simulink model "AnalysisSimAP"  (R2016a)
settings: Solver=VariableStepAuto  StartTime=0.0  StopTime=5  RelTol=1e-3
values from neighbouring files (symbols this model uses):
  C = -C*[1, -1]    [RobustnessAnalysisAP.m]    (also in RobustnessAnalysis_MIL9490.m = -[1; 1]*C*[1, -1])
  GeriFDsysPID2_IO = NdofwActSens(okeep,ikeep,AEC6,ModeShape,FEM,Vmps,aeroProp,massProp,     coeffdataPIDfull,actdata,sensdata)    [GenerateGeriModelAP.m]    (also in RobustnessAnalysisAP.m = P; RobustnessAnalysis_MIL9490.m = P)
  Vinf = Vinfs    [RobustnessAnalysisAP.m]    (also in RobustnessAnalysis_MIL9490.m; example_geri.mat = [25 26 27 28 29 30 31 32 33 34 35 36 ... (21 elements, 1x21))
undefined symbols (not defined in the file or in its folder): K
libraries: simulink_extras x7, cstblocks x5, dspsigattribs x4
settings Model: Creator=Julian  LastModifiedBy=juliant
settings GRTTargetCC: GeneratePreprocessorConditionals=Use local settings

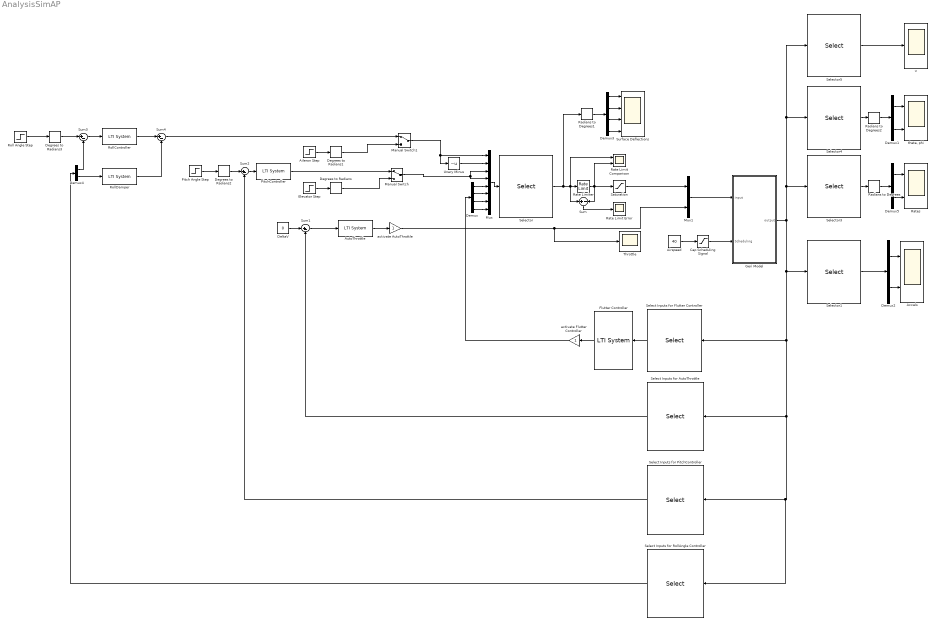
== system AnalysisSimAP ==
  Accels : Scope  NumInputPorts=2
  Aileron Step : Step  Time=3  After=0  SampleTime=0
  Airspeed : Constant  Value=40
  AutoThrottle : cstblocks/LTI System  sys=AutoThrottle  IC=[]
  Cap Scheduling Signal : Saturate  UpperLimit=45  LowerLimit=25
  Degrees to Radians{,1..3} (4 alike) : simulink_extras/Transformations/Degrees to Radians
  DeltaV : Constant  Value=0
  Demux : Demux  Outputs=[1 1 1 1]
  Demux1 : Demux  Outputs=2
  Demux2 : Demux  Outputs=[3 3]
  Demux3 : Demux  Outputs=[2 2 2 2]
  Demux4 : Demux  Outputs=2
  Demux5 : Demux  Outputs=2
  Elevator Step : Step  SampleTime=0
  Flutter Controller : cstblocks/LTI System  sys=-C  IC=[]
  Geri Model : Subsystem
  Manual Switch : ManualSwitch
  Manual Switch1 : ManualSwitch
  Mux : Mux  Inputs=8
  Mux1 : Mux  Inputs=[8 1]
  Pitch Angle Step : Step  Time=0.5  After=10  SampleTime=0
  PitchController : cstblocks/LTI System  sys=PitchController  IC=[]
  Radians to Degrees : simulink_extras/Transformations/Radians to Degrees
  Radians to Degrees1 : simulink_extras/Transformations/Radians to Degrees
  Radians to Degrees2 : simulink_extras/Transformations/Radians to Degrees
  Rate Limit Comparison : Scope  NumInputPorts=2
  Rate Limit Error : Scope
  Rate Limiter : RateLimiter  RisingSlewLimit=30/180*pi  FallingSlewLimit=-30/180*pi  SampleTimeMode=inherited
  Rates : Scope  NumInputPorts=2
  Roll Angle Step : Step  Time=2  After=20  SampleTime=0
  RollController : cstblocks/LTI System  sys=RollController  IC=[]
  RollDamper : cstblocks/LTI System  sys=RollDamper  IC=[]
  Saturation : Saturate  UpperLimit=30/180*pi  LowerLimit=-30/180*pi
  Select Inputs for AutoThrottle : Selector  InputPortWidth=11  IndexOptions=Index vector (dialog)  Indices=1  OutputSizes=1
  Select Inputs for Flutter Controller : Selector  InputPortWidth=11  IndexOptions=Index vector (dialog)  Indices=4:11  OutputSizes=1
  Select Inputs for PitchController : Selector  InputPortWidth=11  IndexOptions=Index vector (dialog)  Indices=2  OutputSizes=1
  Select Inputs for RollAngle Controller : Selector  InputPortWidth=11  IndexOptions=Index vector (dialog)  Indices=[3 5]  OutputSizes=1
  Selector : Selector  InputPortWidth=8  IndexOptions=Index vector (dialog)  Indices=[5 6 1 2 3 4 7 8]  OutputSizes=1
  Selector1 : Selector  InputPortWidth=11  IndexOptions=Index vector (dialog)  Indices=[11 7 10 9 6 8]  OutputSizes=1
  Selector3 : Selector  InputPortWidth=11  IndexOptions=Index vector (dialog)  Indices=[4 5]  OutputSizes=1
  Selector4 : Selector  InputPortWidth=11  IndexOptions=Index vector (dialog)  Indices=[2 3]  OutputSizes=1
  Selector5 : Selector  InputPortWidth=11  IndexOptions=Index vector (dialog)  Indices=[1]  OutputSizes=1
  Sum : Sum  Inputs=+-
  Sum{1..4} (4 alike) : Sum  Inputs=|+-
  Surface Deflections : Scope  NumInputPorts=4
  Throttle : Scope
  Unary Minus : UnaryMinus
  activate AutoThrottle : Gain
  activate Flutter Controller : Gain
  "theta, phi" : Scope  NumInputPorts=2
  u : Scope
  wires:
  Cap Scheduling Signal/1 -> Geri Model/2(Scheduling)
  Airspeed/1 -> Cap Scheduling Signal/1
  Mux/1 -> Selector/1
  Flutter Controller/1 -> activate Flutter Controller/1
  Demux/4 -> Mux/8
  Demux/3 -> Mux/7
  Demux/2 -> Mux/6
  Demux/1 -> Mux/5
  Manual Switch/1 -> Mux/3, Mux/4
  Aileron Step/1 -> Degrees to Radians1/1
  Manual Switch1/1 -> Mux/1, Unary Minus/1
  Selector3/1 -> Radians to Degrees/1
  Geri Model/1(output) -> Selector5/1, Selector4/1, Selector3/1, Selector1/1, Select Inputs for RollAngle Controller/1, Select Inputs for PitchController/1, Select Inputs for AutoThrottle/1, Select Inputs for Flutter Controller/1
  Selector1/1 -> Demux2/1
  Demux2/1 -> Accels/1
  Demux2/2 -> Accels/2
  activate Flutter Controller/1 -> Demux/1
  Radians to Degrees/1 -> Demux5/1
  Radians to Degrees1/1 -> Demux3/1
  Demux3/1 -> Surface Deflections/1
  Demux3/3 -> Surface Deflections/3
  Demux3/2 -> Surface Deflections/2
  Demux3/4 -> Surface Deflections/4
  Saturation/1 -> Mux1/1
  Rate Limiter/1 -> Saturation/1, Sum/2, Rate Limit Comparison/2
  Sum/1 -> Rate Limit Error/1
  Select Inputs for Flutter Controller/1 -> Flutter Controller/1
  AutoThrottle/1 -> activate AutoThrottle/1
  Select Inputs for AutoThrottle/1 -> Sum1/2
  Sum1/1 -> AutoThrottle/1
  DeltaV/1 -> Sum1/1
  Elevator Step/1 -> Degrees to Radians/1
  Pitch Angle Step/1 -> Degrees to Radians2/1
  Sum2/1 -> PitchController/1
  Select Inputs for PitchController/1 -> Sum2/2
  PitchController/1 -> Manual Switch/1
  Sum4/1 -> Manual Switch1/1
  Sum3/1 -> RollController/1
  Roll Angle Step/1 -> Degrees to Radians3/1
  Select Inputs for RollAngle Controller/1 -> Demux4/1
  Degrees to Radians1/1 -> Manual Switch1/2
  Degrees to Radians/1 -> Manual Switch/2
  Degrees to Radians2/1 -> Sum2/1
  Degrees to Radians3/1 -> Sum3/1
  RollController/1 -> Sum4/1
  RollDamper/1 -> Sum4/2
  Demux4/2 -> RollDamper/1
  Demux4/1 -> Sum3/2
  Selector/1 -> Radians to Degrees1/1, Sum/1, Rate Limit Comparison/1, Rate Limiter/1
  Radians to Degrees2/1 -> Demux1/1
  Selector4/1 -> Radians to Degrees2/1
  Selector5/1 -> u/1
  Demux1/1 -> "theta, phi"/1
  Demux1/2 -> "theta, phi"/2
  Demux5/1 -> Rates/1
  Demux5/2 -> Rates/2
  Unary Minus/1 -> Mux/2
  activate AutoThrottle/1 -> Throttle/1, Mux1/2
  Mux1/1 -> Geri Model/1(input)

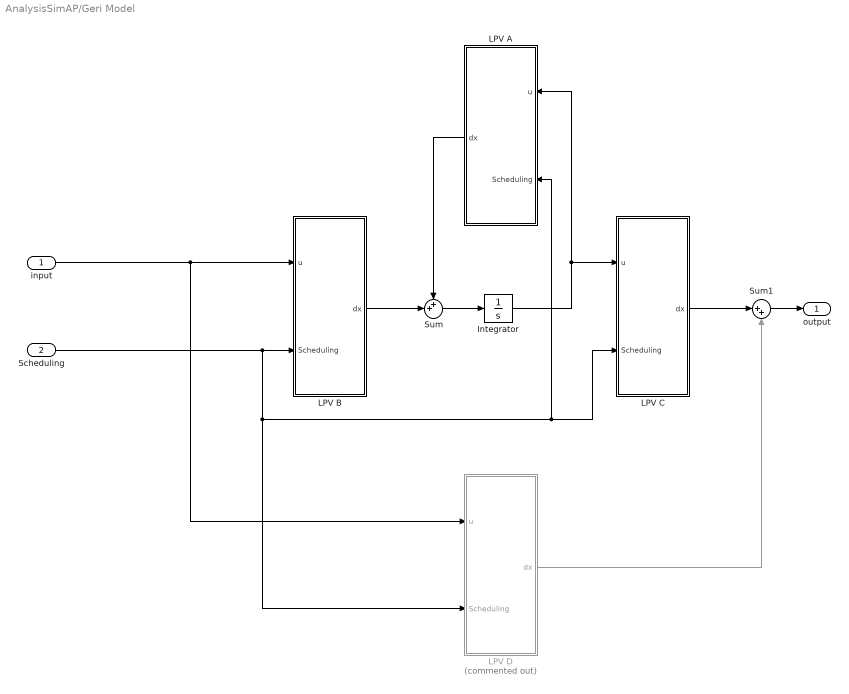
== system AnalysisSimAP/Geri Model ==
  input : Inport
  Scheduling : Inport  Port=2
  Integrator : Integrator  InitialCondition=zeros(size(GeriFDsysPID2_IO.a,1),1)
  LPV A : Subsystem
  LPV B : Subsystem
  LPV C : Subsystem
  LPV D : Subsystem  Commented=on
  Sum : Sum  Inputs=++|
  Sum1 : Sum  Inputs=|++
  output : Outport
  wires:
  LPV C/1(dx) -> Sum1/1
  Sum/1 -> Integrator/1
  Integrator/1 -> LPV C/1(u), LPV A/1(u)
  input/1 -> LPV D/1(u), LPV B/1(u)
  Scheduling/1 -> LPV B/2(Scheduling), LPV D/2(Scheduling), LPV C/2(Scheduling), LPV A/2(Scheduling)
  LPV B/1(dx) -> Sum/2
  LPV A/1(dx) -> Sum/1
  Sum1/1 -> output/1
  LPV D/1(dx) -> Sum1/2

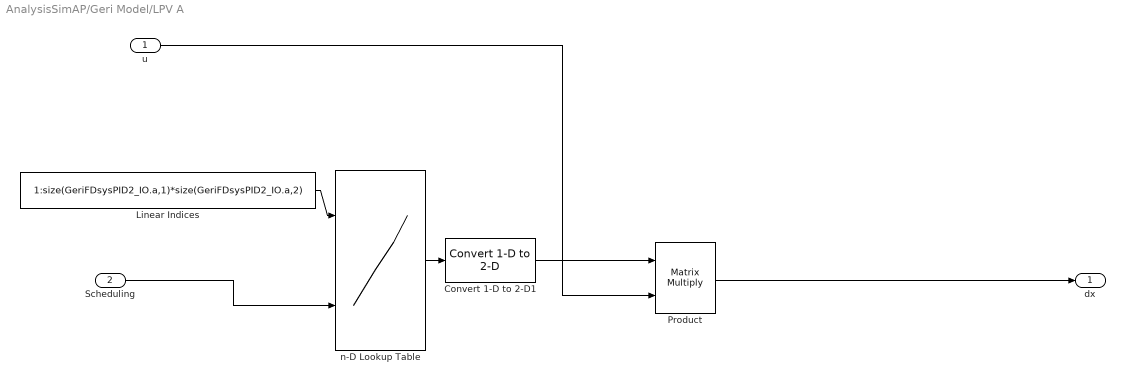
== system AnalysisSimAP/Geri Model/LPV A ==
  u : Inport
  Scheduling : Inport  Port=2
  Convert 1-D to 2-D1 : dspsigattribs/Convert 1-D to 2-D  M=size(GeriFDsysPID2_IO.a,1)  N=size(GeriFDsysPID2_IO.a,2)  frameBasedOut=off
  Linear Indices : Constant  Value=1:size(GeriFDsysPID2_IO.a,1)*size(GeriFDsysPID2_IO.a,2)
  Product : Product  Multiplication=Matrix(*)
  n-D Lookup Table : Lookup_n-D  BreakpointsForDimension1=1:size(GeriFDsysPID2_IO.a,1)*size(GeriFDsysPID2_IO.a,2)  BreakpointsForDimension2=Vinf  BreakpointsForDimension3=K.Parameter.q2.GridData  BreakpointsForDimension4=K.Parameter.q3.GridData  BreakpointsForDimension5=q3.GridData  BeginIndexSearchUsingPreviousIndexResult=on  Table=reshape(GeriFDsysPID2_IO.a,[size(GeriFDsysPID2_IO.a,1)*size(GeriFDsysPID2_IO.a,2), numel(Vinf)])  ExtrapMethod=Clip  UseLastTableValue=on  InternalRulePriority=Speed  RndMeth=Simplest  InputSameDT=on
  dx : Outport
  wires:
  Scheduling/1 -> n-D Lookup Table/2
  u/1 -> Product/2
  Linear Indices/1 -> n-D Lookup Table/1
  Convert 1-D to 2-D1/1 -> Product/1
  n-D Lookup Table/1 -> Convert 1-D to 2-D1/1
  Product/1 -> dx/1

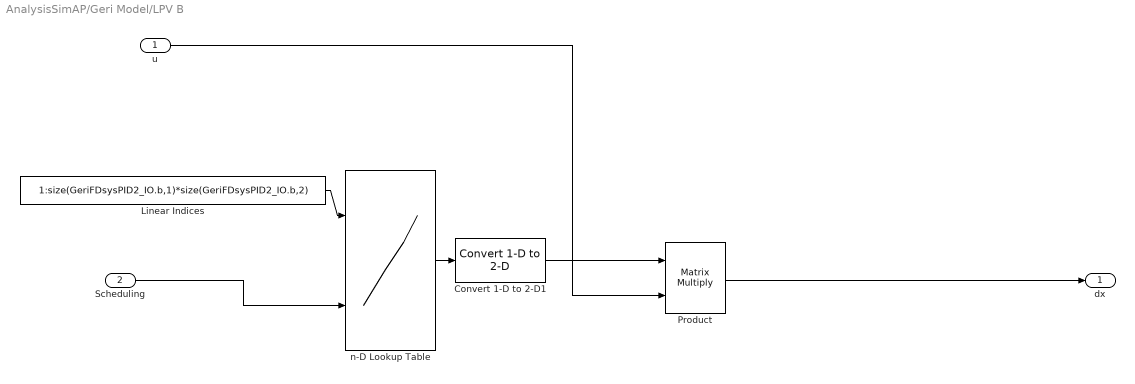
== system AnalysisSimAP/Geri Model/LPV B ==
  u : Inport
  Scheduling : Inport  Port=2
  Convert 1-D to 2-D1 : dspsigattribs/Convert 1-D to 2-D  M=size(GeriFDsysPID2_IO.b,1)  N=size(GeriFDsysPID2_IO.b,2)  frameBasedOut=off
  Linear Indices : Constant  Value=1:size(GeriFDsysPID2_IO.b,1)*size(GeriFDsysPID2_IO.b,2)
  Product : Product  Multiplication=Matrix(*)
  n-D Lookup Table : Lookup_n-D  BreakpointsForDimension1=1:size(GeriFDsysPID2_IO.b,1)*size(GeriFDsysPID2_IO.b,2)  BreakpointsForDimension2=Vinf  BreakpointsForDimension3=K.Parameter.q2.GridData  BreakpointsForDimension4=K.Parameter.q3.GridData  BreakpointsForDimension5=q3.GridData  BeginIndexSearchUsingPreviousIndexResult=on  Table=reshape(GeriFDsysPID2_IO.b,[size(GeriFDsysPID2_IO.b,1)*size(GeriFDsysPID2_IO.b,2), numel(Vinf)])  ExtrapMethod=Clip  UseLastTableValue=on  InternalRulePriority=Speed  RndMeth=Simplest  InputSameDT=on
  dx : Outport
  wires:
  Product/1 -> dx/1
  n-D Lookup Table/1 -> Convert 1-D to 2-D1/1
  Convert 1-D to 2-D1/1 -> Product/1
  Linear Indices/1 -> n-D Lookup Table/1
  u/1 -> Product/2
  Scheduling/1 -> n-D Lookup Table/2

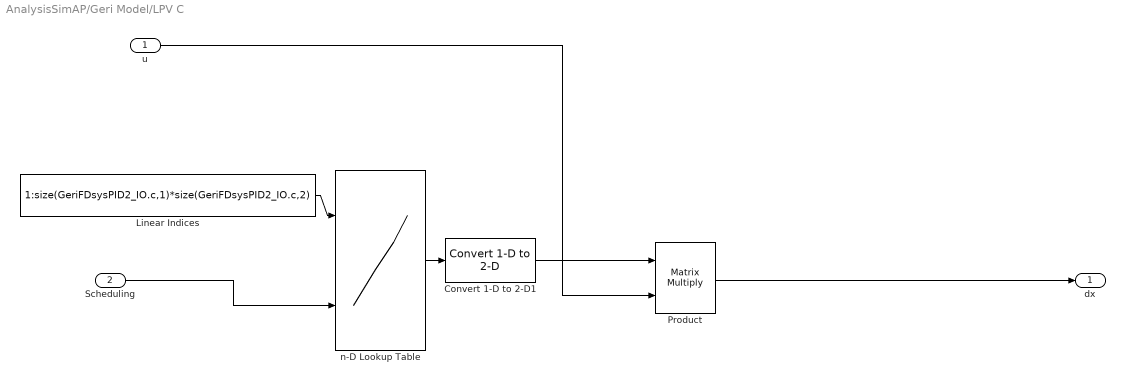
== system AnalysisSimAP/Geri Model/LPV C ==
  u : Inport
  Scheduling : Inport  Port=2
  Convert 1-D to 2-D1 : dspsigattribs/Convert 1-D to 2-D  M=size(GeriFDsysPID2_IO.c,1)  N=size(GeriFDsysPID2_IO.c,2)  frameBasedOut=off
  Linear Indices : Constant  Value=1:size(GeriFDsysPID2_IO.c,1)*size(GeriFDsysPID2_IO.c,2)
  Product : Product  Multiplication=Matrix(*)
  n-D Lookup Table : Lookup_n-D  BreakpointsForDimension1=1:size(GeriFDsysPID2_IO.c,1)*size(GeriFDsysPID2_IO.c,2)  BreakpointsForDimension2=Vinf  BreakpointsForDimension3=K.Parameter.q2.GridData  BreakpointsForDimension4=K.Parameter.q3.GridData  BreakpointsForDimension5=q3.GridData  Table=reshape(GeriFDsysPID2_IO.c,[size(GeriFDsysPID2_IO.c,1)*size(GeriFDsysPID2_IO.c,2), numel(Vinf)])  ExtrapMethod=Clip  UseLastTableValue=on  InternalRulePriority=Speed  RndMeth=Simplest  InputSameDT=on
  dx : Outport
  wires:
  Scheduling/1 -> n-D Lookup Table/2
  u/1 -> Product/2
  Linear Indices/1 -> n-D Lookup Table/1
  Convert 1-D to 2-D1/1 -> Product/1
  n-D Lookup Table/1 -> Convert 1-D to 2-D1/1
  Product/1 -> dx/1

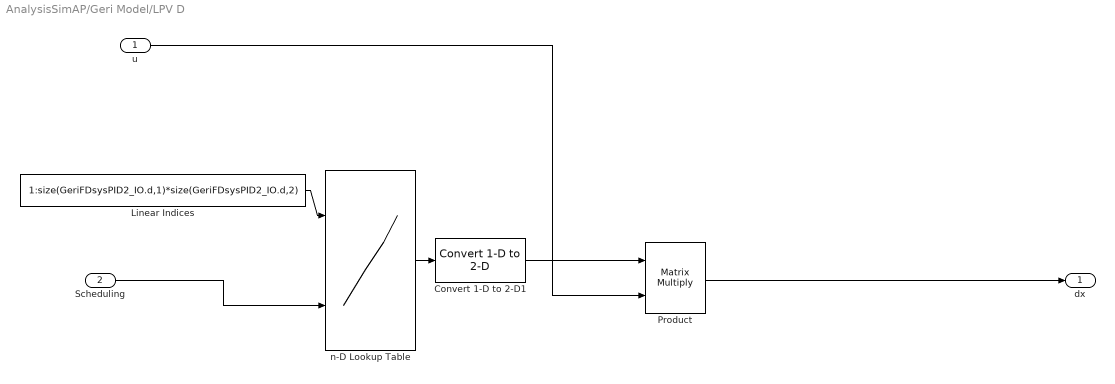
== system AnalysisSimAP/Geri Model/LPV D ==
  u : Inport
  Scheduling : Inport  Port=2
  Convert 1-D to 2-D1 : dspsigattribs/Convert 1-D to 2-D  M=size(GeriFDsysPID2_IO.d,1)  N=size(GeriFDsysPID2_IO.d,2)  frameBasedOut=off
  Linear Indices : Constant  Value=1:size(GeriFDsysPID2_IO.d,1)*size(GeriFDsysPID2_IO.d,2)
  Product : Product  Multiplication=Matrix(*)
  n-D Lookup Table : Lookup_n-D  BreakpointsForDimension1=1:size(GeriFDsysPID2_IO.d,1)*size(GeriFDsysPID2_IO.d,2)  BreakpointsForDimension2=Vinf  BreakpointsForDimension3=K.Parameter.q2.GridData  BreakpointsForDimension4=K.Parameter.q3.GridData  BreakpointsForDimension5=q3.GridData  Table=reshape(GeriFDsysPID2_IO.d,[size(GeriFDsysPID2_IO.d,1)*size(GeriFDsysPID2_IO.d,2), numel(Vinf)])  ExtrapMethod=Clip  UseLastTableValue=on  InternalRulePriority=Speed  RndMeth=Simplest  InputSameDT=on
  dx : Outport
  wires:
  Product/1 -> dx/1
  n-D Lookup Table/1 -> Convert 1-D to 2-D1/1
  Convert 1-D to 2-D1/1 -> Product/1
  Linear Indices/1 -> n-D Lookup Table/1
  u/1 -> Product/2
  Scheduling/1 -> n-D Lookup Table/2
